simulink model "PMSM_FOC_Speed_Closedloop(old)"  (R2022a)
settings: Solver=FixedStepDiscrete  StartTime=0.0  StopTime=1  FixedStep=0.00001  RelTol=1e-3
model workspace (MAT data in the model file):
  K = 0
libraries: simulink x3, slpidlib x3, spsDCVoltageSourceLib x1, spsPermanentMagnetSynchronousMachineLib x1, spsTwoLevelConverterLib x1, spspowerguiLib x1
settings Model: Creator=A  LastModifiedBy=A

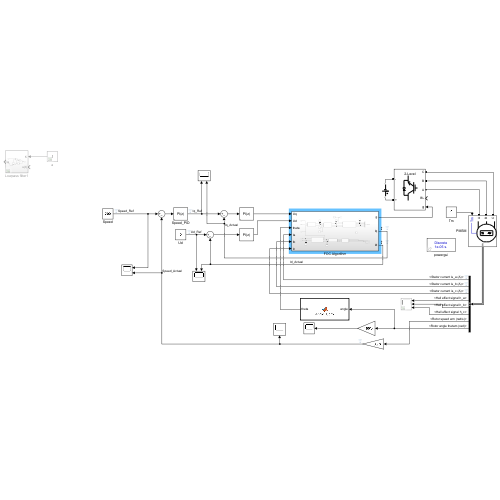
[thumbnail: Simulink's stored preview of the top-level diagram]
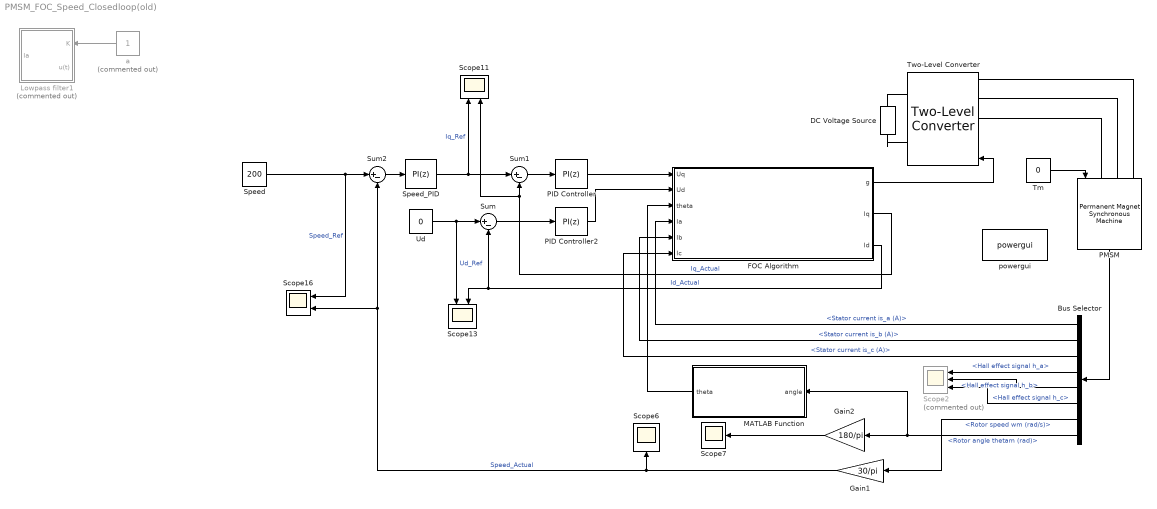
== system PMSM_FOC_Speed_Closedloop(old) ==
  Bus Selector : BusSelector  OutputSignals=Stator current is_a (A),Stator current is_b (A),Stator current is_c (A),Hall effect signal h_a,Hall effect signal h_b,Hall effect signal h_c,Rotor speed wm (rad/s),Rotor angle thetam (rad)
  DC Voltage Source : spsDCVoltageSourceLib/DC Voltage Source  Amplitude=12  Measurements=None
  FOC Algorithm : Subsystem
  Gain1 : Gain  Gain=30/pi
  Gain2 : Gain  Gain=180/pi
  Lowpass filter1 : Subsystem  Commented=on
  MATLAB Function : MATLAB Function  TreatAsAtomicUnit=on
  PID Controller : slpidlib/PID Controller  Controller=PI  Form=Parallel  TimeDomain=Discrete-time  UseExternalTs=off  SampleTime=-1  IntegratorMethod=Forward Euler  FilterMethod=Forward Euler  ControllerParametersSource=internal  P=2  I=0.2  UseKiTs=off  D=0  N=100  UseFilter=on  TunerSelectOption=Transfer Function Based (PID Tuner App)  InitialConditionSource=internal  InitialConditionForIntegrator=0  InitialConditionForFilter=0  DifferentiatorICPrevScaledInput=0  ExternalReset=none  TrackingMode=off  Kt=1  LimitOutput=off  SatLimitsSource=internal  UpperSaturationLimit=inf  LowerSaturationLimit=-inf  LinearizeAsGain=on  AntiWindupMode=none  Kb=1  POutMin=[]  POutMax=[]  IOutMin=[]  IOutMax=[]  DOutMin=[]  DOutMax=[]  NOutMin=[]  NOutMax=[]  SumOutMin=[]  SumOutMax=[]  SaturationOutMin=[]  SaturationOutMax=[]  PParamMin=[]  PParamMax=[]  IParamMin=[]  IParamMax=[]  DParamMin=[]  DParamMax=[]  NParamMin=[]  NParamMax=[]  KbParamMin=[]  KbParamMax=[]  KtParamMin=[]  KtParamMax=[]  KbOutMin=[]  KbOutMax=[]  KtOutMin=[]  KtOutMax=[]  IntegratorOutMin=[]  IntegratorOutMax=[]  FilterOutMin=[]  FilterOutMax=[]  SumI1OutMin=[]  SumI1OutMax=[]  SumI2OutMin=[]  SumI2OutMax=[]  SumI3OutMin=[]  SumI3OutMax=[]  SumI4OutMin=[]  SumI4OutMax=[]  SumDOutMin=[]  SumDOutMax=[]  DifferentiatorOutMin=[]  DifferentiatorOutMax=[]  FilterDiffOutCoefMin=[]  FilterDiffOutCoefMax=[]  ReciprocalOutMin=[]  ReciprocalOutMax=[]  SumDenOutMin=[]  SumDenOutMax=[]  SumNumOutMin=[]  SumNumOutMax=[]  DivideOutMin=[]  DivideOutMax=[]  UdiffTsProdOutMin=[]  UdiffTsProdOutMax=[]  NTsProdOutMin=[]  NTsProdOutMax=[]  UintegralTsProdOutMin=[]  UintegralTsProdOutMax=[]  UngainTsProdOutMin=[]  UngainTsProdOutMax=[]  IntegratorContinuousStateAttributes=''  IntegratorStateMustResolveToSignalObject=off  IntegratorRTWStateStorageClass=Auto  FilterContinuousStateAttributes=''  FilterStateMustResolveToSignalObject=off  FilterRTWStateStorageClass=Auto  ParallelPVariant=InternalParameters  IdealPVariant=Disabled  IVariant=InternalParameters  DVariant=Disabled  IntegratorVariant=Discrete  SatVariant=Disabled  AWVariant=Passthrough  PCopyVariant=Disabled  TRVariant=Disabled  FdbkBlocksVariant=Forward  IdealPFdbkVariant=Disabled  SatFdbkVariant=Disabled  DerivativeFilterVariant=Disabled  NVariant=Disabled  NCopyVariant=Disabled_SignalSpec  FilterICVariant=Disabled  IntegratorICVariant=InternalICs  ExternalResetVariant=Disabled  TRSumVariant=Passthrough  SumFdbkVariant=Disabled  SumVariant=Sum_PI  TsampFilterVariant=InternalTs  TsampNgainVariant=Passthrough  TsampIntegralVariant=Passthrough  ExternalSaturationOutDataTypeStr=Inherit: Same as second input  aMode=0
  PID Controller2 : slpidlib/PID Controller  Controller=PI  Form=Parallel  TimeDomain=Discrete-time  UseExternalTs=off  SampleTime=-1  IntegratorMethod=Forward Euler  FilterMethod=Forward Euler  ControllerParametersSource=internal  P=1  I=0.2  UseKiTs=off  D=0  N=100  UseFilter=on  TunerSelectOption=Transfer Function Based (PID Tuner App)  InitialConditionSource=internal  InitialConditionForIntegrator=0  InitialConditionForFilter=0  DifferentiatorICPrevScaledInput=0  ExternalReset=none  TrackingMode=off  Kt=1  LimitOutput=off  SatLimitsSource=internal  UpperSaturationLimit=inf  LowerSaturationLimit=-inf  LinearizeAsGain=on  AntiWindupMode=none  Kb=1  POutMin=[]  POutMax=[]  IOutMin=[]  IOutMax=[]  DOutMin=[]  DOutMax=[]  NOutMin=[]  NOutMax=[]  SumOutMin=[]  SumOutMax=[]  SaturationOutMin=[]  SaturationOutMax=[]  PParamMin=[]  PParamMax=[]  IParamMin=[]  IParamMax=[]  DParamMin=[]  DParamMax=[]  NParamMin=[]  NParamMax=[]  KbParamMin=[]  KbParamMax=[]  KtParamMin=[]  KtParamMax=[]  KbOutMin=[]  KbOutMax=[]  KtOutMin=[]  KtOutMax=[]  IntegratorOutMin=[]  IntegratorOutMax=[]  FilterOutMin=[]  FilterOutMax=[]  SumI1OutMin=[]  SumI1OutMax=[]  SumI2OutMin=[]  SumI2OutMax=[]  SumI3OutMin=[]  SumI3OutMax=[]  SumI4OutMin=[]  SumI4OutMax=[]  SumDOutMin=[]  SumDOutMax=[]  DifferentiatorOutMin=[]  DifferentiatorOutMax=[]  FilterDiffOutCoefMin=[]  FilterDiffOutCoefMax=[]  ReciprocalOutMin=[]  ReciprocalOutMax=[]  SumDenOutMin=[]  SumDenOutMax=[]  SumNumOutMin=[]  SumNumOutMax=[]  DivideOutMin=[]  DivideOutMax=[]  UdiffTsProdOutMin=[]  UdiffTsProdOutMax=[]  NTsProdOutMin=[]  NTsProdOutMax=[]  UintegralTsProdOutMin=[]  UintegralTsProdOutMax=[]  UngainTsProdOutMin=[]  UngainTsProdOutMax=[]  IntegratorContinuousStateAttributes=''  IntegratorStateMustResolveToSignalObject=off  IntegratorRTWStateStorageClass=Auto  FilterContinuousStateAttributes=''  FilterStateMustResolveToSignalObject=off  FilterRTWStateStorageClass=Auto  ParallelPVariant=InternalParameters  IdealPVariant=Disabled  IVariant=InternalParameters  DVariant=Disabled  IntegratorVariant=Discrete  SatVariant=Disabled  AWVariant=Passthrough  PCopyVariant=Disabled  TRVariant=Disabled  FdbkBlocksVariant=Forward  IdealPFdbkVariant=Disabled  SatFdbkVariant=Disabled  DerivativeFilterVariant=Disabled  NVariant=Disabled  NCopyVariant=Disabled_SignalSpec  FilterICVariant=Disabled  IntegratorICVariant=InternalICs  ExternalResetVariant=Disabled  TRSumVariant=Passthrough  SumFdbkVariant=Disabled  SumVariant=Sum_PI  TsampFilterVariant=InternalTs  TsampNgainVariant=Passthrough  TsampIntegralVariant=Passthrough  ExternalSaturationOutDataTypeStr=Inherit: Same as second input  aMode=0
  PMSM : spsPermanentMagnetSynchronousMachineLib/Permanent Magnet Synchronous Machine  NbPhases=3  FluxDistribution=Sinusoidal  RotorType=Round  MechanicalLoad=Torque Tm  PresetModel=No  ShowDetailedParameters=on  MeasurementBus=off  Resistance=0.0485  Inductance=8.5e-3  dqInductances=[8.5e-3,8.5e-3]  La=0.000395  MachineConstant=Flux linkage established by magnets (V.s)  Flux=0.1194  VoltageCst=43.3135  TorqueCst=0.3582  Flat=120  Mechanical=[0.0027 0.0004924 2 0]  PolePairs=4  InitialConditions=[0,0, 0,0]  InitialConditions5ph=[0 0 0 0 0 0]  RefAngle=Aligned with phase A axis (original Park)  IterativeDiscreteModel=Trapezoidal non iterative  TsBlock=-1  TsPowergui=0
  Scope11 : Scope  NumInputPorts=2
  Scope13 : Scope  NumInputPorts=2
  Scope16 : Scope  NumInputPorts=2
  Scope2 : Scope  Commented=on  NumInputPorts=3
  Scope6 : Scope
  Scope7 : Scope
  Speed : Constant  Value=200
  Speed_PID : slpidlib/PID Controller  Controller=PI  Form=Parallel  TimeDomain=Discrete-time  UseExternalTs=off  SampleTime=-1  IntegratorMethod=Forward Euler  FilterMethod=Forward Euler  ControllerParametersSource=internal  P=1  I=20  UseKiTs=off  D=0  N=100  UseFilter=on  TunerSelectOption=Transfer Function Based (PID Tuner App)  InitialConditionSource=internal  InitialConditionForIntegrator=0  InitialConditionForFilter=0  DifferentiatorICPrevScaledInput=0  ExternalReset=none  TrackingMode=off  Kt=1  LimitOutput=off  SatLimitsSource=internal  UpperSaturationLimit=inf  LowerSaturationLimit=-inf  LinearizeAsGain=on  AntiWindupMode=none  Kb=1  POutMin=[]  POutMax=[]  IOutMin=[]  IOutMax=[]  DOutMin=[]  DOutMax=[]  NOutMin=[]  NOutMax=[]  SumOutMin=[]  SumOutMax=[]  SaturationOutMin=[]  SaturationOutMax=[]  PParamMin=[]  PParamMax=[]  IParamMin=[]  IParamMax=[]  DParamMin=[]  DParamMax=[]  NParamMin=[]  NParamMax=[]  KbParamMin=[]  KbParamMax=[]  KtParamMin=[]  KtParamMax=[]  KbOutMin=[]  KbOutMax=[]  KtOutMin=[]  KtOutMax=[]  IntegratorOutMin=[]  IntegratorOutMax=[]  FilterOutMin=[]  FilterOutMax=[]  SumI1OutMin=[]  SumI1OutMax=[]  SumI2OutMin=[]  SumI2OutMax=[]  SumI3OutMin=[]  SumI3OutMax=[]  SumI4OutMin=[]  SumI4OutMax=[]  SumDOutMin=[]  SumDOutMax=[]  DifferentiatorOutMin=[]  DifferentiatorOutMax=[]  FilterDiffOutCoefMin=[]  FilterDiffOutCoefMax=[]  ReciprocalOutMin=[]  ReciprocalOutMax=[]  SumDenOutMin=[]  SumDenOutMax=[]  SumNumOutMin=[]  SumNumOutMax=[]  DivideOutMin=[]  DivideOutMax=[]  UdiffTsProdOutMin=[]  UdiffTsProdOutMax=[]  NTsProdOutMin=[]  NTsProdOutMax=[]  UintegralTsProdOutMin=[]  UintegralTsProdOutMax=[]  UngainTsProdOutMin=[]  UngainTsProdOutMax=[]  IntegratorContinuousStateAttributes=''  IntegratorStateMustResolveToSignalObject=off  IntegratorRTWStateStorageClass=Auto  FilterContinuousStateAttributes=''  FilterStateMustResolveToSignalObject=off  FilterRTWStateStorageClass=Auto  ParallelPVariant=InternalParameters  IdealPVariant=Disabled  IVariant=InternalParameters  DVariant=Disabled  IntegratorVariant=Discrete  SatVariant=Disabled  AWVariant=Passthrough  PCopyVariant=Disabled  TRVariant=Disabled  FdbkBlocksVariant=Forward  IdealPFdbkVariant=Disabled  SatFdbkVariant=Disabled  DerivativeFilterVariant=Disabled  NVariant=Disabled  NCopyVariant=Disabled_SignalSpec  FilterICVariant=Disabled  IntegratorICVariant=InternalICs  ExternalResetVariant=Disabled  TRSumVariant=Passthrough  SumFdbkVariant=Disabled  SumVariant=Sum_PI  TsampFilterVariant=InternalTs  TsampNgainVariant=Passthrough  TsampIntegralVariant=Passthrough  ExternalSaturationOutDataTypeStr=Inherit: Same as second input  aMode=0
  Sum : Sum  Inputs=|+-
  Sum1 : Sum  Inputs=|+-
  Sum2 : Sum  Inputs=|+-
  Tm : Constant  Value=0
  Two-Level Converter : spsTwoLevelConverterLib/Two-Level Converter  ModelType=Switching devices  Ron=1e-3  Rs=1e6  Cs=inf  Vforward=[0,0]  Ron_Diode=1e-3  Rs_Diode=1e6  Cs_Diode=inf  Vf_Diode=1e-3  Rs_CurrentSource=inf  Ron_ACsource=1e-3
      settings: SourceProductBaseCode=PS
  Ud : Constant  Value=0
  a : Constant  Commented=on
  powergui : spspowerguiLib/powergui  Priority=1  SimulationMode=Discrete  SampleTime=0.00001  frequency=60  Iterations=50  frequencyindice=0  Pbase=100e6  ErrMax=1e-4  UnitsV=kV  UnitsW=MW  buscounter=0  FunctionMessages=off  echomessages=off  EnableUseOfTLC=off  CurrentSourceSwitches=off  DisableSnubberDevices=off  DisableRonSwitches=off  DisableVfSwitches=off  DisplayEquations=off  AutomaticDiscreteSolvers=off  SolverType=Tustin/Backward Euler (TBE)  Interpol=off  ExternalGateDelay=off  methode=off  Ts=100  x0status=blocks  SPID=on  SwTol=0  HookPort=off  NonlinearTolerance=1e-4  nMaxIteration=100  ContinueOnMaxIteration=off  RestoreLinks=warning  ResistiveCurrentMeasurement=off  Frange=[0:2:500]  Ylog=off  Xlog=on  ShowGrid=off  save=off  variable=ZData  structure=0  ZoomFFT=off  StartTime=0.0  cycles=1  DisplayStyle=1  fundamental=60  FreqAxis=off  MaxFrequency=1000  frequencyindicesteady=1  RmsSteady=1  display=off
  wires:
  PMSM/1 -> Bus Selector/1
  Bus Selector/4 -> Scope2/1  "<Hall effect signal h_a>"
  Bus Selector/5 -> Scope2/2  "<Hall effect signal h_b>"
  Bus Selector/6 -> Scope2/3  "<Hall effect signal h_c>"
  Bus Selector/7 -> Gain1/1  "<Rotor speed wm (rad/s)>"
  Tm/1 -> PMSM/1
  Bus Selector/8 -> MATLAB Function/1(angle), Gain2/1  "<Rotor angle thetam (rad)>"
  Gain2/1 -> Scope7/1
  PID Controller/1 -> FOC Algorithm/1(Uq)
  Bus Selector/1 -> FOC Algorithm/4(Ia)  "<Stator current is_a (A)>"
  Bus Selector/2 -> FOC Algorithm/5(Ib)  "<Stator current is_b (A)>"
  Bus Selector/3 -> FOC Algorithm/6(Ic)  "<Stator current is_c (A)>"
  FOC Algorithm/1(g) -> Two-Level Converter/1
  a/1 -> Lowpass filter1/1(K)
  MATLAB Function/1(theta) -> FOC Algorithm/3(theta)
  Speed/1 -> Scope16/1, Sum2/1  "Speed_Ref"
  Ud/1 -> Sum/1, Scope13/1  "Ud_Ref"
  Speed_PID/1 -> Scope11/1, Sum1/1  "Iq_Ref"
  Sum2/1 -> Speed_PID/1
  Sum1/1 -> PID Controller/1
  Gain1/1 -> Sum2/2, Scope16/2, Scope6/1  "Speed_Actual"
  FOC Algorithm/2(Iq) -> Scope11/2, Sum1/2  "Iq_Actual"
  FOC Algorithm/3(Id) -> Sum/2, Scope13/2  "Id_Actual"
  Sum/1 -> PID Controller2/1
  PID Controller2/1 -> FOC Algorithm/2(Ud)
  connections:
  Two-Level Converter/LConn1 -- PMSM/LConn1
  Two-Level Converter/LConn2 -- PMSM/LConn2
  PMSM/LConn3 -- Two-Level Converter/LConn3
  DC Voltage Source/RConn1 -- Two-Level Converter/RConn1
  DC Voltage Source/LConn1 -- Two-Level Converter/RConn2

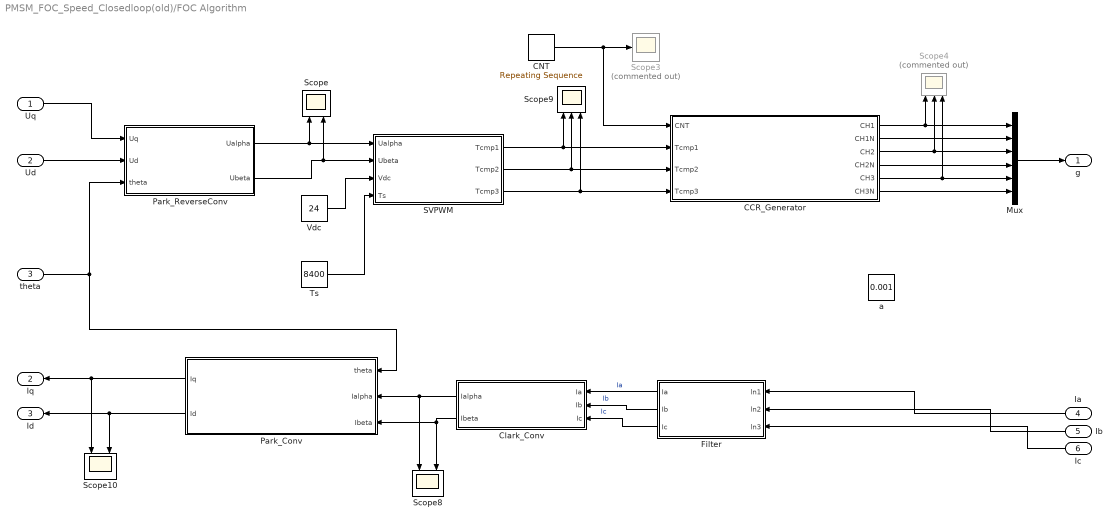
== system PMSM_FOC_Speed_Closedloop(old)/FOC Algorithm ==
  Uq : Inport
  Ud : Inport  Port=2
  theta : Inport  Port=3
  Ia : Inport  Port=4
  Ib : Inport  Port=5
  Ic : Inport  Port=6
  CCR_Generator : MATLAB Function  TreatAsAtomicUnit=on
  CNT : simulink/Sources/Repeating Sequence  rep_seq_t=[0 1/200 1/100]  rep_seq_y=[0 4200 0]
  Clark_Conv : Subsystem
  Filter : Subsystem  Variant=on
  Mux : Mux  Inputs=6
  Park_Conv : Subsystem
  Park_ReverseConv : Subsystem
  SVPWM : Subsystem
  Scope : Scope  NumInputPorts=2
  Scope10 : Scope  NumInputPorts=2
  Scope3 : Scope  Commented=on
  Scope4 : Scope  Commented=on  NumInputPorts=3
  Scope8 : Scope  NumInputPorts=2
  Scope9 : Scope  NumInputPorts=3
  Ts : Constant  Value=8400
  Vdc : Constant  Value=24
  a : Constant  Value=0.001
  g : Outport
  Iq : Outport  Port=2
  Id : Outport  Port=3
  wires:
  Uq/1 -> Park_ReverseConv/1(Uq)
  SVPWM/3(Tcmp3) -> CCR_Generator/4(Tcmp3), Scope9/3
  Clark_Conv/1(Ialpha) -> Park_Conv/2(Ialpha), Scope8/1
  CCR_Generator/3(CH2) -> Mux/3, Scope4/2
  SVPWM/2(Tcmp2) -> CCR_Generator/3(Tcmp2), Scope9/2
  CCR_Generator/2(CH1N) -> Mux/2
  theta/1 -> Park_Conv/1(theta), Park_ReverseConv/3(theta)
  Ts/1 -> SVPWM/4(Ts)
  CCR_Generator/5(CH3) -> Mux/5, Scope4/3
  SVPWM/1(Tcmp1) -> CCR_Generator/2(Tcmp1), Scope9/1
  Clark_Conv/2(Ibeta) -> Park_Conv/3(Ibeta), Scope8/2
  CCR_Generator/4(CH2N) -> Mux/4
  Park_ReverseConv/1(Ualpha) -> SVPWM/1(Ualpha), Scope/1
  CCR_Generator/6(CH3N) -> Mux/6
  Mux/1 -> g/1
  Park_ReverseConv/2(Ubeta) -> Scope/2, SVPWM/2(Ubeta)
  CNT/1 -> Scope3/1, CCR_Generator/1(CNT)
  Park_Conv/2(Id) -> Scope10/2, Id/1
  CCR_Generator/1(CH1) -> Mux/1, Scope4/1
  Vdc/1 -> SVPWM/3(Vdc)
  Ud/1 -> Park_ReverseConv/2(Ud)
  Park_Conv/1(Iq) -> Scope10/1, Iq/1
  Filter/1(Ia) -> Clark_Conv/1(Ia)  "Ia"
  Filter/2(Ib) -> Clark_Conv/2(Ib)  "Ib"
  Filter/3(Ic) -> Clark_Conv/3(Ic)  "Ic"
  Ia/1 -> Filter/1(ln1)
  Ib/1 -> Filter/2(ln2)
  Ic/1 -> Filter/3(ln3)

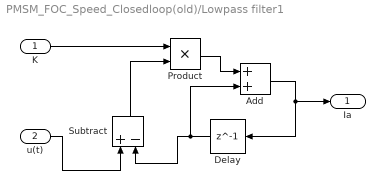
== system PMSM_FOC_Speed_Closedloop(old)/Lowpass filter1 ==
  K : Inport
  u(t) : Inport  Port=2
  Add : Sum
  Delay : Delay  DelayLength=1
  Product : Product
  Subtract : Sum  Inputs=+-
  Ia : Outport
  wires:
  Add/1 -> Ia/1, Delay/1
  Product/1 -> Add/1
  Subtract/1 -> Product/2
  Delay/1 -> Subtract/2, Add/2
  K/1 -> Product/1
  u(t)/1 -> Subtract/1

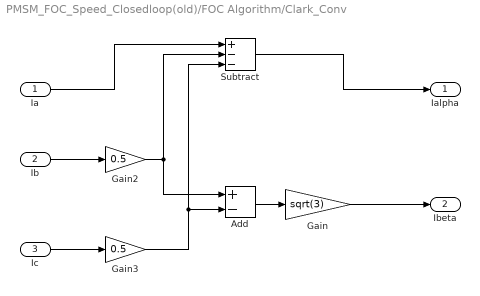
== system PMSM_FOC_Speed_Closedloop(old)/FOC Algorithm/Clark_Conv ==
  Ia : Inport
  Ib : Inport  Port=2
  Ic : Inport  Port=3
  Add : Sum  Inputs=+-
  Gain : Gain  Gain=sqrt(3)
  Gain2 : Gain  Gain=0.5
  Gain3 : Gain  Gain=0.5
  Subtract : Sum  Inputs=+--
  Ialpha : Outport
  Ibeta : Outport  Port=2
  wires:
  Ia/1 -> Subtract/1
  Ib/1 -> Gain2/1
  Add/1 -> Gain/1
  Gain/1 -> Ibeta/1
  Ic/1 -> Gain3/1
  Gain2/1 -> Subtract/2, Add/1
  Gain3/1 -> Subtract/3, Add/2
  Subtract/1 -> Ialpha/1

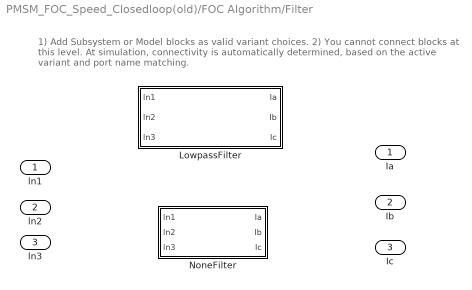
== system PMSM_FOC_Speed_Closedloop(old)/FOC Algorithm/Filter ==
  note: 1) Add Subsystem or Model blocks as valid variant choices.
      | 2) You cannot connect blocks at this level. At simulation, connectivity is automatically
      | determined, based on the active variant and port name matching.
  ln1 : Inport
  ln2 : Inport  Port=2
  ln3 : Inport  Port=3
  LowpassFilter : Subsystem  VariantControl=K==1
  NoneFilter : Subsystem  VariantControl=K==0
  Ia : Outport
  Ib : Outport  Port=2
  Ic : Outport  Port=3

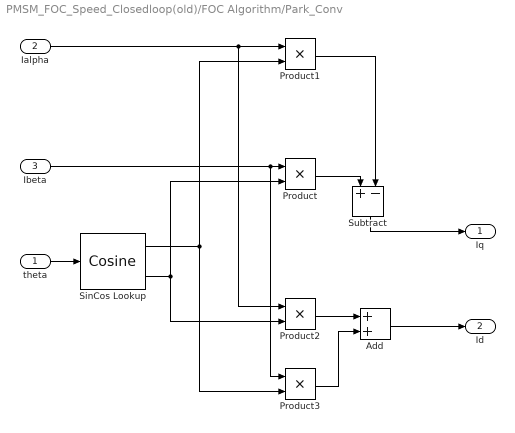
== system PMSM_FOC_Speed_Closedloop(old)/FOC Algorithm/Park_Conv ==
  theta : Inport
  Ialpha : Inport  Port=2
  Ibeta : Inport  Port=3
  Add : Sum
  Product{,1..3} (4 alike) : Product
  SinCos Lookup : simulink/Lookup Tables/Cosine  Formula=sin(2*pi*u) and cos(2*pi*u)  NumDataPoints=(2^5)+1  OutputWordLength=16  InternalRulePriority=Speed
      settings: SourceProductBaseCode=SL
  Subtract : Sum  Inputs=+-
  Iq : Outport
  Id : Outport  Port=2
  wires:
  Ialpha/1 -> Product1/1, Product2/1
  Ibeta/1 -> Product3/1, Product/1
  theta/1 -> SinCos Lookup/1
  SinCos Lookup/2 -> Product2/2, Product/2
  SinCos Lookup/1 -> Product3/2, Product1/2
  Product1/1 -> Subtract/2
  Subtract/1 -> Iq/1
  Product/1 -> Subtract/1
  Product2/1 -> Add/1
  Product3/1 -> Add/2
  Add/1 -> Id/1

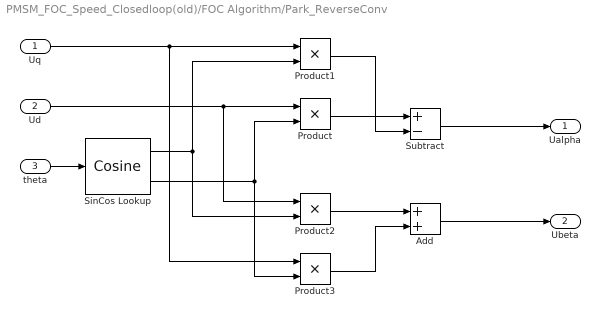
== system PMSM_FOC_Speed_Closedloop(old)/FOC Algorithm/Park_ReverseConv ==
  Uq : Inport
  Ud : Inport  Port=2
  theta : Inport  Port=3
  Add : Sum
  Product{,1..3} (4 alike) : Product
  SinCos Lookup : simulink/Lookup Tables/Cosine  Formula=sin(2*pi*u) and cos(2*pi*u)  NumDataPoints=(2^5)+1  OutputWordLength=16  InternalRulePriority=Speed
      settings: SourceProductBaseCode=SL
  Subtract : Sum  Inputs=+-
  Ualpha : Outport
  Ubeta : Outport  Port=2
  wires:
  Uq/1 -> Product3/1, Product1/1
  theta/1 -> SinCos Lookup/1
  Ud/1 -> Product2/1, Product/1
  SinCos Lookup/2 -> Product3/2, Product/2
  Product/1 -> Subtract/1
  SinCos Lookup/1 -> Product2/2, Product1/2
  Product1/1 -> Subtract/2
  Subtract/1 -> Ualpha/1
  Product2/1 -> Add/1
  Product3/1 -> Add/2
  Add/1 -> Ubeta/1

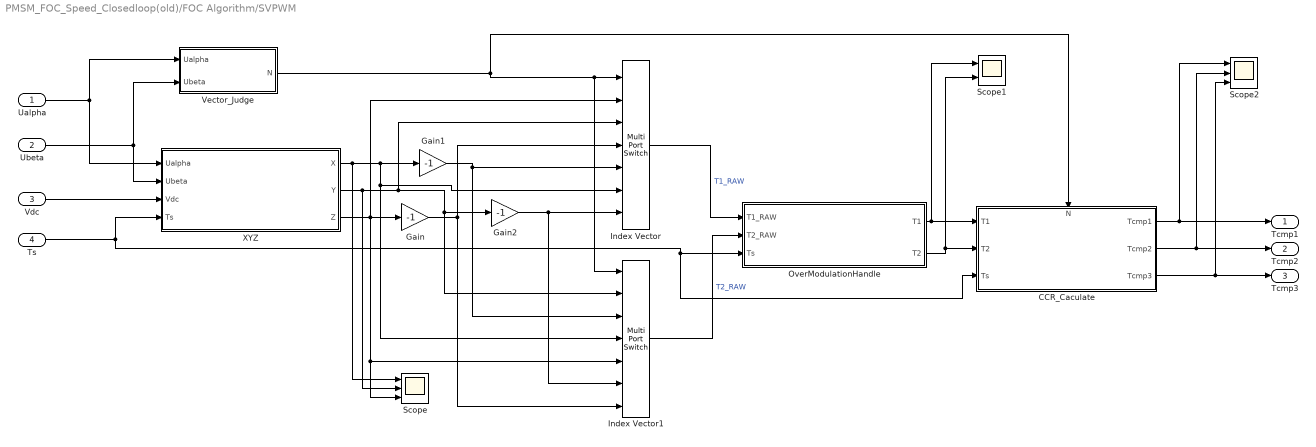
== system PMSM_FOC_Speed_Closedloop(old)/FOC Algorithm/SVPWM ==
  Ualpha : Inport
  Ubeta : Inport  Port=2
  Vdc : Inport  Port=3
  Ts : Inport  Port=4
  CCR_Caculate : Subsystem
      settings: PortSchema="{\"entries\":[{\"content\":{\"sides\":[{\"content\":{\"connectorIds\":[\"In1\",\"In2\",\"In3\"]},\"type\":\"ConnectorPlacement.EquallySpacedRectSide\",\"uuid\":\"41d89106-695f-4d7e-9c99-c52170b99868\"},{\"content\":{\"connectorIds\":[\"Out1\",\"Out2\",\"Out3\"],\"side\":\"RIGHT\"},\"type\":\"ConnectorPlacement.EquallySpacedRectSide\",\"uuid\":\"0fa1e6b9-7088-4c16-9dd3-c016449aae3e\"},{\"content\":{\"connectorIds\":[\"In4\"],\"side\":\"TOP\"},\"type\":\"ConnectorPlacement.EquallySpacedRectSide\",\"uuid\":\"6b702c00-29ab-49c7-a344-eb6fce3368af\"}]},\"type\":\"ConnectorPlacement.EquallySpacedConnector\",\"uuid\":\"c2f99839-550c-47c5-98fa-a115626cfb71\"}],\"packageUris\":[\"http://schema.mathworks.com/mf0/Connector/R2020b\"],\"version\":\"1.0\"}"
  Gain : Gain  Gain=-1
  Gain1 : Gain  Gain=-1
  Gain2 : Gain  Gain=-1
  Index Vector : MultiPortSwitch  Inputs=6  SaturateOnIntegerOverflow=off  InputSameDT=off
  Index Vector1 : MultiPortSwitch  Inputs=6  SaturateOnIntegerOverflow=off  InputSameDT=off
  OverModulationHandle : MATLAB Function  TreatAsAtomicUnit=on
  Scope : Scope  NumInputPorts=3
  Scope1 : Scope  NumInputPorts=2
  Scope2 : Scope  NumInputPorts=3
  Vector_Judge : Subsystem
  XYZ : Subsystem
  Tcmp1 : Outport
  Tcmp2 : Outport  Port=2
  Tcmp3 : Outport  Port=3
  wires:
  Ualpha/1 -> Vector_Judge/1(Ualpha), XYZ/1(Ualpha)
  Ubeta/1 -> Vector_Judge/2(Ubeta), XYZ/2(Ubeta)
  Vdc/1 -> XYZ/3(Vdc)
  Ts/1 -> CCR_Caculate/3(Ts), OverModulationHandle/3(Ts), XYZ/4(Ts)
  Vector_Judge/1(N) -> Index Vector1/1, Index Vector/1, CCR_Caculate/4(N)
  Index Vector1/1 -> OverModulationHandle/2(T2_RAW)  "T2_RAW"
  XYZ/3(Z) -> Scope/3, Index Vector1/5, Index Vector/2, Gain/1
  XYZ/2(Y) -> Scope/2, Index Vector1/2, Gain2/1, Index Vector/3
  Gain/1 -> Index Vector1/7, Index Vector/4
  XYZ/1(X) -> Scope/1, Index Vector1/4, Index Vector/6, Gain1/1
  Gain1/1 -> Index Vector1/3, Index Vector/5
  Gain2/1 -> Index Vector1/6, Index Vector/7
  Index Vector/1 -> OverModulationHandle/1(T1_RAW)  "T1_RAW"
  OverModulationHandle/1(T1) -> CCR_Caculate/1(T1), Scope1/1
  OverModulationHandle/2(T2) -> Scope1/2, CCR_Caculate/2(T2)
  CCR_Caculate/1(Tcmp1) -> Tcmp1/1, Scope2/1
  CCR_Caculate/2(Tcmp2) -> Tcmp2/1, Scope2/2
  CCR_Caculate/3(Tcmp3) -> Tcmp3/1, Scope2/3

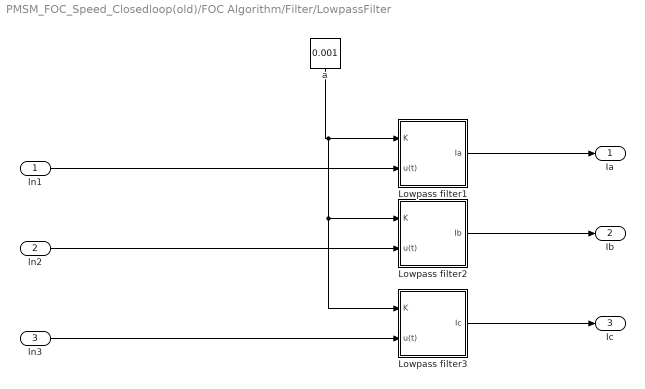
== system PMSM_FOC_Speed_Closedloop(old)/FOC Algorithm/Filter/LowpassFilter ==
  ln1 : Inport
  ln2 : Inport  Port=2
  ln3 : Inport  Port=3
  Lowpass filter1 : Subsystem
  Lowpass filter2 : Subsystem
  Lowpass filter3 : Subsystem
  a : Constant  Value=0.001
  Ia : Outport
  Ib : Outport  Port=2
  Ic : Outport  Port=3
  wires:
  ln2/1 -> Lowpass filter2/2(u(t))
  a/1 -> Lowpass filter3/1(K), Lowpass filter2/1(K), Lowpass filter1/1(K)
  ln1/1 -> Lowpass filter1/2(u(t))
  Lowpass filter1/1(Ia) -> Ia/1
  Lowpass filter2/1(Ib) -> Ib/1
  Lowpass filter3/1(Ic) -> Ic/1
  ln3/1 -> Lowpass filter3/2(u(t))

== system PMSM_FOC_Speed_Closedloop(old)/FOC Algorithm/Filter/NoneFilter ==
  ln1 : Inport
  ln2 : Inport  Port=2
  ln3 : Inport  Port=3
  Ia : Outport
  Ib : Outport  Port=2
  Ic : Outport  Port=3
  wires:
  ln1/1 -> Ia/1
  ln2/1 -> Ib/1
  ln3/1 -> Ic/1

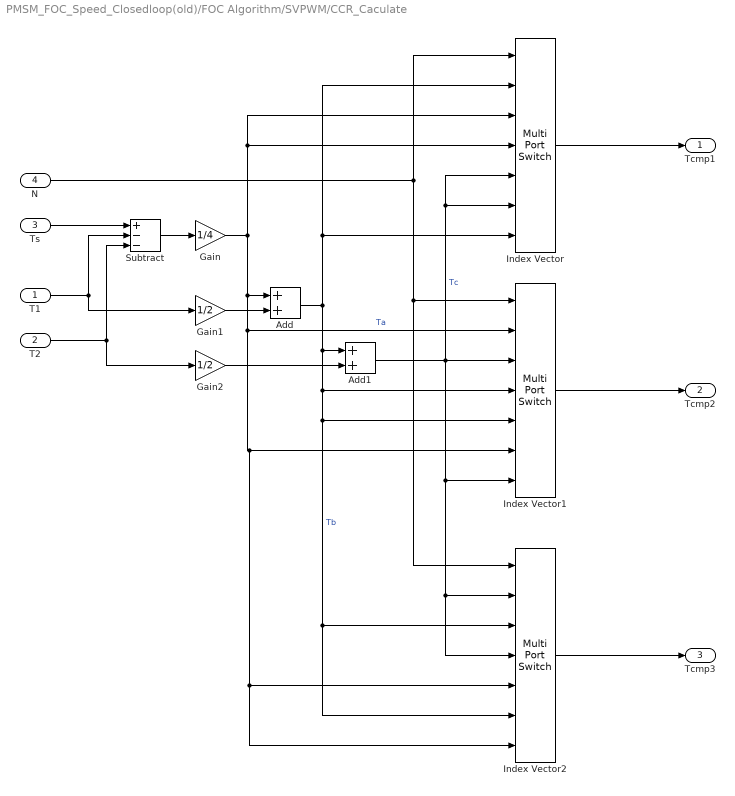
== system PMSM_FOC_Speed_Closedloop(old)/FOC Algorithm/SVPWM/CCR_Caculate ==
  T1 : Inport
  T2 : Inport  Port=2
  Ts : Inport  Port=3
  N : Inport  Port=4
  Add : Sum
  Add1 : Sum
  Gain : Gain  Gain=1/4
  Gain1 : Gain  Gain=1/2
  Gain2 : Gain  Gain=1/2
  Index Vector : MultiPortSwitch  Inputs=6  SaturateOnIntegerOverflow=off  InputSameDT=off
  Index Vector1 : MultiPortSwitch  Inputs=6  SaturateOnIntegerOverflow=off  InputSameDT=off
  Index Vector2 : MultiPortSwitch  Inputs=6  SaturateOnIntegerOverflow=off  InputSameDT=off
  Subtract : Sum  Inputs=+--
  Tcmp1 : Outport
  Tcmp2 : Outport  Port=2
  Tcmp3 : Outport  Port=3
  wires:
  Ts/1 -> Subtract/1
  T1/1 -> Gain1/1, Subtract/2
  T2/1 -> Gain2/1, Subtract/3
  Subtract/1 -> Gain/1
  Gain/1 -> Index Vector2/7, Index Vector2/5, Index Vector1/6, Index Vector1/2, Add/1, Index Vector/4, Index Vector/3  "Ta"
  Gain1/1 -> Add/2
  Add/1 -> Index Vector1/5, Index Vector2/6, Index Vector2/3, Index Vector1/4, Add1/1, Index Vector/7, Index Vector/2  "Tb"
  Gain2/1 -> Add1/2
  Add1/1 -> Index Vector2/4, Index Vector2/2, Index Vector1/7, Index Vector1/3, Index Vector/6, Index Vector/5  "Tc"
  N/1 -> Index Vector2/1, Index Vector1/1, Index Vector/1
  Index Vector/1 -> Tcmp1/1
  Index Vector1/1 -> Tcmp2/1
  Index Vector2/1 -> Tcmp3/1

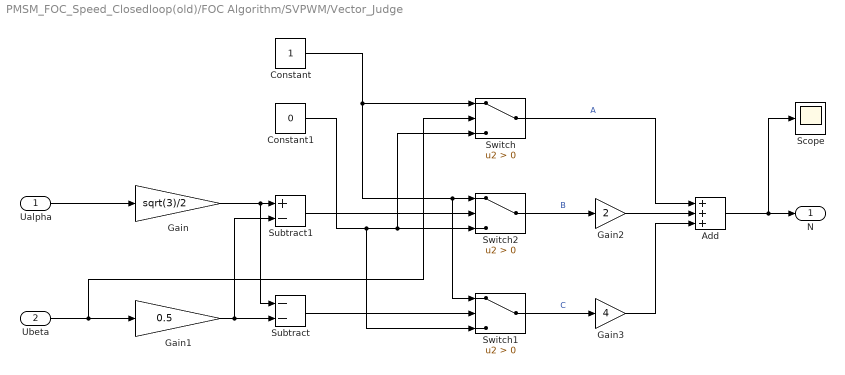
== system PMSM_FOC_Speed_Closedloop(old)/FOC Algorithm/SVPWM/Vector_Judge ==
  Ualpha : Inport
  Ubeta : Inport  Port=2
  Add : Sum  Inputs=+++
  Constant : Constant
  Constant1 : Constant  Value=0
  Gain : Gain  Gain=sqrt(3)/2
  Gain1 : Gain  Gain=0.5
  Gain2 : Gain  Gain=2
  Gain3 : Gain  Gain=4
  Scope : Scope
  Subtract : Sum  Inputs=--
  Subtract1 : Sum  Inputs=+-
  Switch : Switch  Criteria=u2 > Threshold  SaturateOnIntegerOverflow=off  InputSameDT=off
  Switch1 : Switch  Criteria=u2 > Threshold  SaturateOnIntegerOverflow=off  InputSameDT=off
  Switch2 : Switch  Criteria=u2 > Threshold  SaturateOnIntegerOverflow=off  InputSameDT=off
  N : Outport
  wires:
  Ualpha/1 -> Gain/1
  Ubeta/1 -> Gain1/1, Switch/2
  Switch/1 -> Add/1  "A"
  Switch1/1 -> Gain3/1  "C"
  Constant1/1 -> Switch2/3, Switch/3, Switch1/3
  Constant/1 -> Switch2/1, Switch1/1, Switch/1
  Switch2/1 -> Gain2/1  "B"
  Gain3/1 -> Add/3
  Add/1 -> Scope/1, N/1
  Gain2/1 -> Add/2
  Gain/1 -> Subtract/1, Subtract1/1
  Gain1/1 -> Subtract/2, Subtract1/2
  Subtract1/1 -> Switch2/2
  Subtract/1 -> Switch1/2

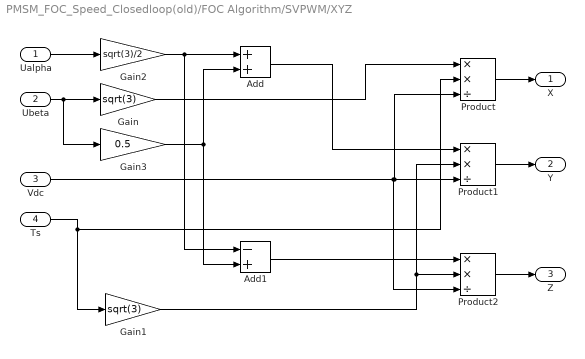
== system PMSM_FOC_Speed_Closedloop(old)/FOC Algorithm/SVPWM/XYZ ==
  Ualpha : Inport
  Ubeta : Inport  Port=2
  Vdc : Inport  Port=3
  Ts : Inport  Port=4
  Add : Sum
  Add1 : Sum  Inputs=-+
  Gain : Gain  Gain=sqrt(3)
  Gain1 : Gain  Gain=sqrt(3)
  Gain2 : Gain  Gain=sqrt(3)/2
  Gain3 : Gain  Gain=0.5
  Product : Product  Inputs=**/
  Product1 : Product  Inputs=**/
  Product2 : Product  Inputs=**/
  X : Outport
  Y : Outport  Port=2
  Z : Outport  Port=3
  wires:
  Ualpha/1 -> Gain2/1
  Gain/1 -> Product/1
  Ubeta/1 -> Gain3/1, Gain/1
  Ts/1 -> Product/2, Gain1/1
  Vdc/1 -> Product1/3, Product/3, Product2/3
  Product/1 -> X/1
  Gain2/1 -> Add1/1, Add/1
  Gain3/1 -> Add/2, Add1/2
  Add/1 -> Product1/1
  Gain1/1 -> Product2/2, Product1/2
  Product1/1 -> Y/1
  Add1/1 -> Product2/1
  Product2/1 -> Z/1

== system PMSM_FOC_Speed_Closedloop(old)/FOC Algorithm/Filter/LowpassFilter/Lowpass filter1 ==
  K : Inport
  u(t) : Inport  Port=2
  Add : Sum
  Delay : Delay  DelayLength=1
  Product : Product
  Subtract : Sum  Inputs=+-
  Ia : Outport
  wires:
  Add/1 -> Ia/1, Delay/1
  Product/1 -> Add/1
  Subtract/1 -> Product/2
  Delay/1 -> Subtract/2, Add/2
  K/1 -> Product/1
  u(t)/1 -> Subtract/1

== system PMSM_FOC_Speed_Closedloop(old)/FOC Algorithm/Filter/LowpassFilter/Lowpass filter2 ==
  K : Inport
  u(t) : Inport  Port=2
  Add : Sum
  Delay : Delay  DelayLength=1
  Product : Product
  Subtract : Sum  Inputs=+-
  Ib : Outport
  wires:
  u(t)/1 -> Subtract/1
  K/1 -> Product/1
  Delay/1 -> Add/2, Subtract/2
  Subtract/1 -> Product/2
  Product/1 -> Add/1
  Add/1 -> Delay/1, Ib/1

== system PMSM_FOC_Speed_Closedloop(old)/FOC Algorithm/Filter/LowpassFilter/Lowpass filter3 ==
  K : Inport
  u(t) : Inport  Port=2
  Add : Sum
  Delay : Delay  DelayLength=1
  Product : Product
  Subtract : Sum  Inputs=+-
  Ic : Outport
  wires:
  Add/1 -> Ic/1, Delay/1
  Product/1 -> Add/1
  Subtract/1 -> Product/2
  Delay/1 -> Subtract/2, Add/2
  K/1 -> Product/1
  u(t)/1 -> Subtract/1

== matlab function PMSM_FOC_Speed_Closedloop(old)/FOC Algorithm/CCR_Generator ==
  data: CNT input; Tcmp1 input; Tcmp2 input; Tcmp3 input; CH1 output; CH1N output; CH2 output; CH2N output; CH3 output; CH3N output
function[CH1,CH1N,CH2,CH2N,CH3,CH3N] = CCR_Generator(CNT,Tcmp1, Tcmp2, Tcmp3)

if (CNT<Tcmp1)
    CH1=0;
    CH1N=1;
else
    CH1=1;
    CH1N=0;
end
if (CNT<Tcmp2)
    CH2=0;
    CH2N=1;
else
    CH2=1;
    CH2N=0;
end
if (CNT<Tcmp3)
    CH3=0;
    CH3N=1;
else
    CH3=1;
    CH3N=0;
end
end

== matlab function PMSM_FOC_Speed_Closedloop(old)/FOC Algorithm/SVPWM/OverModulationHandle ==
  data: T1_RAW input; T2_RAW input; T1 output; T2 output; Ts input
function [T1,T2] = OverModulationHandle(T1_RAW, T2_RAW, Ts)
if((T1_RAW+T2_RAW)>Ts)
    T1=T1_RAW/(T1_RAW+T2_RAW)*Ts;
    T2=T2_RAW/(T1_RAW+T2_RAW)*Ts;
else
    T1=T1_RAW;
    T2=T2_RAW;
end
end

== matlab function PMSM_FOC_Speed_Closedloop(old)/MATLAB Function ==
  data: angle input; theta output
function theta = Angle_Conv(angle)

n=mod(angle,pi)/pi;

theta = n;
